simulink model "srf_pll_arch"  (R2023a)
settings: configuration reference "QuickStart_50024_6_23_9_31_16537" (kept outside this file)
settings Model: DataDictionary=dictionary_srf_pll.sldd  Creator=ASUSTUF  LastModifiedBy=ASUSTUF
settings ConfigSetRef: SourceName=QuickStart_50024_6_23_9_31_16537

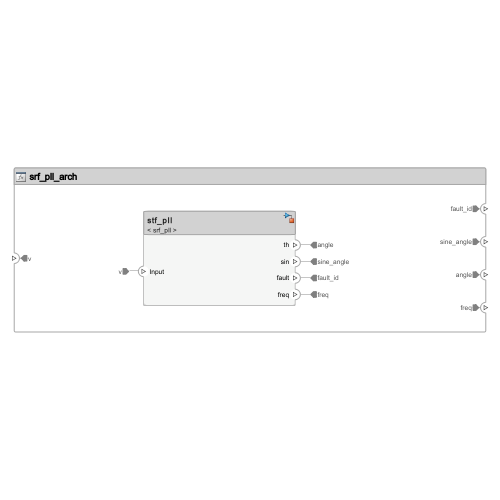
[thumbnail: Simulink's stored preview of the top-level diagram]
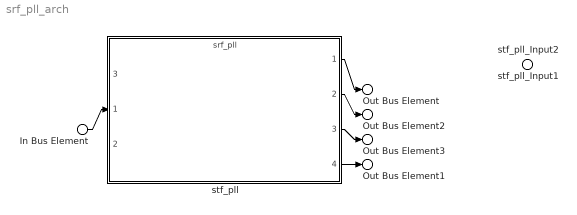
== system srf_pll_arch ==
  In Bus Element : Inport  PortName=v
  stf_pll_Input1 : Inport  Port=2  OutputFunctionCall=on
  stf_pll_Input2 : Inport  Port=3  OutputFunctionCall=on
  stf_pll : ModelReference  ModelNameDialog=srf_pll  SimulationMode=Normal  ScheduleRates=on  ModelReferenceVersion=1.31
      settings: PortSchema="{\"entries\":[{\"content\":{\"headerSize\":38,\"margin\":15,\"minimumSpacing\":25,\"sides\":[{\"content\":{\"connectorIds\":[\"In1\"]},\"type\":\"ConnectorPlacement.EquallySpacedRectSide\",\"uuid\":\"58e1e09c-1481-422c-98e1-11bdc88c978a\"},{\"content\":{\"connectorIds\":[\"Out1\",\"Out2\",\"Out3\",\"Out4\"],\"side\":\"RIGHT\"},\"type\":\"ConnectorPlacement.EquallySpacedRectSide\",\"uuid\":\"f717c870-d9f3-41d0-95bd-1e96e0fd0290\"},{\"content\":{\"side\":\"TOP\"},\"type\":\"ConnectorPlacement.EquallySpacedRectSide\",\"uuid\":\"bca3bf00-b17f-40ff-8364-387dab955bb1\"},{\"content\":{\"connectorIds\":[\"In3\",\"In2\"],\"side\":\"HIDDEN\"},\"type\":\"ConnectorPlacement.EquallySpacedRectSide\",\"uuid\":\"836c40e6-9558-4cc0-9803-e417237341e7\"}]},\"type\":\"ConnectorPlacement.EquallySpacedConnector\",\"uuid\":\"a14bb22f-aea4-41ba-917e-73fe63090ce2\"}],\"packageUris\":[\"http://schema.mathworks.com/mf0/Connector/R2020b\"],\"version\":\"1.0\"}"
  Out Bus Element3 : Outport  PortName=fault_id
  Out Bus Element2 : Outport  Port=2  PortName=sine_angle
  Out Bus Element : Outport  Port=3  PortName=angle
  Out Bus Element1 : Outport  Port=4  PortName=freq
  wires:
  In Bus Element/1 -> stf_pll/1
  stf_pll/3 -> Out Bus Element3/1
  stf_pll/2 -> Out Bus Element2/1
  stf_pll/1 -> Out Bus Element/1
  stf_pll/4 -> Out Bus Element1/1
